simulink model "PSO_MPPT"  (R2018a)
settings: Solver=VariableStepAuto  StartTime=0.0  StopTime=10  FixedStep=1  RelTol=1e-3
libraries: powerlib x9, powerlib_meascontrol x2, re_lib x1
settings Model: Creator=Rodney Tan  LastModifiedBy=hp
settings SolverCC: ZeroCrossAlgorithm=Adaptive  AlgebraicLoopSolver=LineSearch
settings OptimizationCC: LifeSpan=inf
settings DebuggingCC: MaxConsecutiveZCsMsg=none  MaskedZcDiagnostic=none  IgnoredZcDiagnostic=none  SFUnexpectedBacktrackingDiag=warning  SFNoUnconditionalDefaultTransitionDiag=warning  SFExecutionAtInitializationDiag=none
settings CodeAppCC: StateflowObjectComments=on
settings GRTTargetCC: TargetLangStandard=C89/C90 (ANSI)  GeneratePreprocessorConditionals=Disable all
settings ConfigComp: CovMetricSettings=dw  CovHtmlReporting=on  CovSaveCumulativeToWorkspaceVar=on  CovSaveSingleToWorkspaceVar=on  CovExternalEMLEnable=off
settings SimscapeCC: SimscapeNormalizeSystem=off

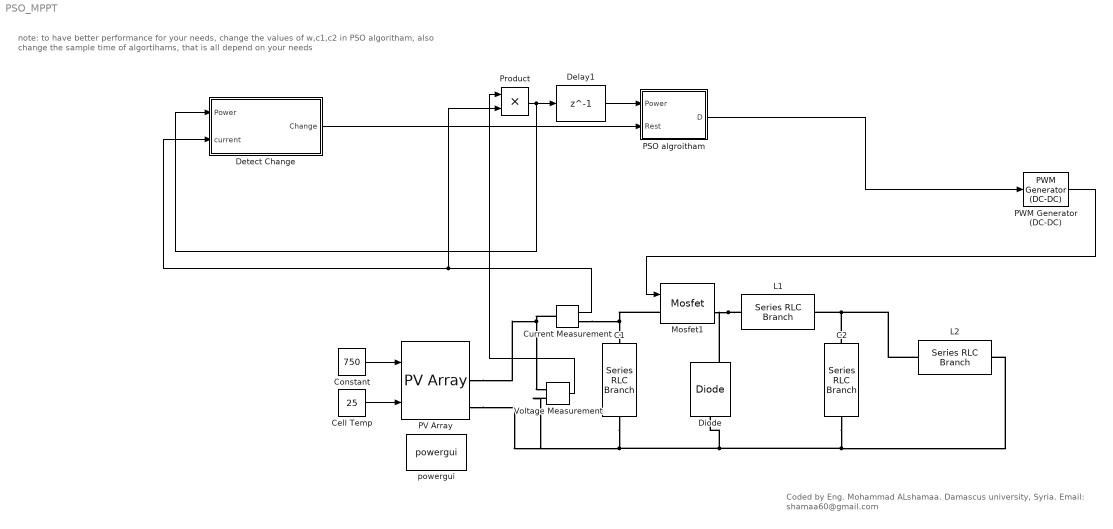
== system PSO_MPPT ==
  note: note: to have better performance for your needs,
      | change the values of w,c1,c2 in PSO algoritham, also change the sample time of algortihams, that is all depend on your needs
  note: Coded by Eng. Mohammad ALshamaa.
      | Damascus university, Syria.
      | Email: shamaa60@gmail.com
  " C2" : powerlib/Elements/Series RLC Branch  LConnTagsString=__new0  RConnTagsString=__new0  BranchType=C  Resistance=0.1  Inductance=1e-3  SetiL0=off  InitialCurrent=0  Capacitance=1000e-6  Setx0=off  InitialVoltage=0  Measurements=None
  C1 : powerlib/Elements/Series RLC Branch  LConnTagsString=__new0  RConnTagsString=__new0  BranchType=C  Resistance=0.1  Inductance=1e-3  SetiL0=off  InitialCurrent=0  Capacitance=1000e-6  Setx0=off  InitialVoltage=0  Measurements=None
  Cell Temp : Constant  Value=25
  Constant : Constant  Value=750
  Current Measurement : powerlib/Measurements/Current Measurement  PhasorSimulation=off  OutputType=Complex  PSBequivalent=0
  Delay1 : Delay  DelayLength=1  InputProcessing=Columns as channels (frame based)
  Detect Change : Subsystem
  Diode : powerlib/Power Electronics/Diode  Ron=0  Lon=0  Vf=0  IC=0  UseSnubber=0  Rs=500  Cs=250e-9  Measurements=on
  L1 : powerlib/Elements/Series RLC Branch  LConnTagsString=__new0  RConnTagsString=__new0  BranchType=L  Resistance=1  Inductance=20e-3  SetiL0=off  InitialCurrent=0  Capacitance=1e-6  Setx0=off  InitialVoltage=0  Measurements=None
  L2 : powerlib/Elements/Series RLC Branch  LConnTagsString=__new0  RConnTagsString=__new0  BranchType=R  Resistance=1  Inductance=10e-3  SetiL0=off  InitialCurrent=0  Capacitance=1e-6  Setx0=off  InitialVoltage=0  Measurements=None
  Mosfet1 : powerlib/Power Electronics/Mosfet  Ron=0  Lon=0  Rd=0  Vfd=0  IC=0  Rs=1e5  Cs=inf  Measurements=on
  PSO algroitham : MATLAB Function  TreatAsAtomicUnit=on  SystemSampleTime=0.05
  PV Array : re_lib/Solar/PV Array  Npar=1  Nser=1  PlotType=array @ 25 deg.C & specified irradiances  S_vec="[ 1000  750  100 ]"  Temp_C_vec="[ 45 25  ]"  ModuleName=1Soltech 1STH-215-P  PlotWhenSelected=off  Pm=213.15  Ncell=60  Voc=36.3  Isc=7.84  Vm=29  Im=7.35  beta_Voc_pc=-0.36099  alpha_Isc_pc=0.102  beta_Voc=-0.13104  alpha_Isc=0.007997  IL=7.8649  I0=2.9259e-10  nI=0.98117  Rsh=313.3991  Rs=0.39383  BAL=off  Tc=1e-6  Tfilter=5e-3
  PWM Generator (DC-DC) : powerlib_meascontrol/Pulse & Signal Generators/PWM Generator (DC-DC)  Fsw=10e3  Ts=0
  Product : Product
  Voltage Measurement : powerlib/Measurements/Voltage Measurement  PhasorSimulation=off  OutputType=Complex  PSBequivalent=0
  powergui : powerlib/powergui  Priority=1  SimulationMode=Continuous  SampleTime=1e-3  frequency=60  Iterations=50  frequencyindice=0  Pbase=100e6  ErrMax=1e-4  UnitsV=kV  UnitsW=MW  buscounter=0  FunctionMessages=off  echomessages=off  EnableUseOfTLC=off  CurrentSourceSwitches=off  DisableSnubberDevices=off  DisableRonSwitches=off  DisableVfSwitches=off  DisplayEquations=off  SolverType=Tustin/Backward Euler (TBE)  Interpol=off  ExternalGateDelay=off  methode=off  Ts=100  x0status=blocks  SPID=off  SwTol=0  HookPort=off  RestoreLinks=warning  ResistiveCurrentMeasurement=off  Frange=[0:2:500]  Ylog=off  Xlog=on  ShowGrid=off  save=off  variable=ZData  structure=0  ZoomFFT=off  StartTime=0.0  cycles=1  DisplayStyle=1  fundamental=60  FreqAxis=off  MaxFrequency=1000  frequencyindicesteady=1  RmsSteady=1  display=off
  wires:
  Cell Temp/1 -> PV Array/2
  Constant/1 -> PV Array/1
  PWM Generator (DC-DC)/1 -> Mosfet1/1
  Voltage Measurement/1 -> Product/1
  Delay1/1 -> PSO algroitham/1(Power)
  PSO algroitham/1(D) -> PWM Generator (DC-DC)/1
  Current Measurement/1 -> Detect Change/2(current), Product/2
  Product/1 -> Detect Change/1(Power), Delay1/1
  Detect Change/1(Change) -> PSO algroitham/2(Rest)
  connections:
  " C2"/LConn1 -- L2/LConn1 -- L1/RConn1
  " C2"/RConn1 -- L2/RConn1 -- Diode/LConn1 -- Voltage Measurement/LConn2 -- PV Array/RConn2 -- C1/RConn1
  L1/LConn1 -- Diode/RConn1 -- Mosfet1/RConn1
  Mosfet1/LConn1 -- Current Measurement/RConn1 -- C1/LConn1
  PV Array/RConn1 -- Current Measurement/LConn1 -- Voltage Measurement/LConn1

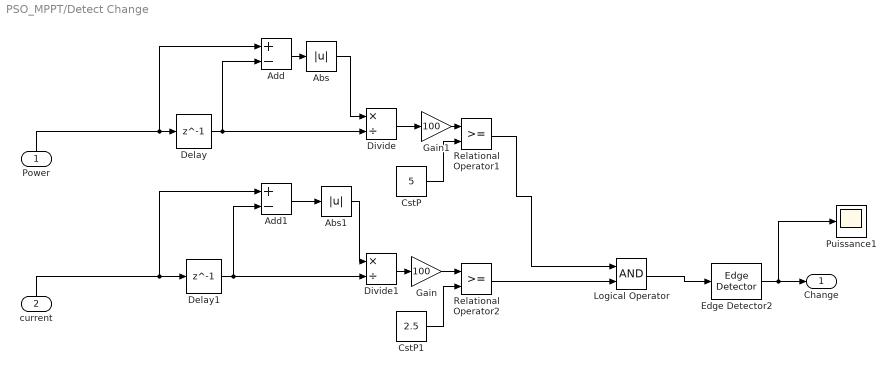
== system PSO_MPPT/Detect Change ==
  Power : Inport
  current : Inport  Port=2
  Abs : Abs
  Abs1 : Abs
  Add : Sum  Inputs=+-
  Add1 : Sum  Inputs=+-
  CstP : Constant  Value=5
  CstP1 : Constant  Value=2.5
  Delay : Delay  DelayLength=1
  Delay1 : Delay  DelayLength=1
  Divide : Product  Inputs=*/
  Divide1 : Product  Inputs=*/
  Edge Detector2 : powerlib_meascontrol/Logic/Edge Detector  model=Rising  ic=0  Ts=0
      settings: SourceProductName=Simscape Power Systems  SourceProductBaseCode=PS
  Gain : Gain  Gain=100
  Gain1 : Gain  Gain=100
  Logical Operator : Logic  AllPortsSameDT=off  OutDataTypeStr=boolean
  Puissance1 : Scope
  Relational Operator1 : RelationalOperator  OutDataTypeStr=boolean  RndMeth=Nearest
  Relational Operator2 : RelationalOperator  OutDataTypeStr=boolean  RndMeth=Nearest
  Change : Outport
  wires:
  Relational Operator1/1 -> Logical Operator/1
  Add/1 -> Abs/1
  Delay/1 -> Divide/2, Add/2
  Power/1 -> Add/1, Delay/1
  Abs/1 -> Divide/1
  CstP/1 -> Relational Operator1/2
  Logical Operator/1 -> Edge Detector2/1
  Delay1/1 -> Add1/2, Divide1/2
  CstP1/1 -> Relational Operator2/2
  current/1 -> Add1/1, Delay1/1
  Abs1/1 -> Divide1/1
  Add1/1 -> Abs1/1
  Relational Operator2/1 -> Logical Operator/2
  Divide1/1 -> Gain/1
  Gain/1 -> Relational Operator2/1
  Divide/1 -> Gain1/1
  Gain1/1 -> Relational Operator1/1
  Edge Detector2/1 -> Puissance1/1, Change/1

== matlab function PSO_MPPT/PSO algroitham ==
  settings: updateMethod=DISCRETE
  data: Power input; D output; Rest input
function D   = fcn(Power, Rest)
persistent particals
persistent pbest
persistent gbest
persistent velocity
persistent Dcurrent
persistent Powerbest
persistent u
persistent gpowerbest
persistent idx
persistent xx
if isempty(xx)
   xx=0; 
end
if isempty(particals) || (Rest==1 && xx==1)
particals=zeros(4,1); 
particals(1)=0.2;
particals(2)=0.3;
particals(3)=0.6;
particals(4)=0.9;
velocity=zeros(4,1)
pbest=zeros(4,1);
Powerbest=zeros(4,1);
gbest=0.5;
Dcurrent=0;
gpowerbest=0;
u=0;
idx=0;
end
if sum(abs(velocity))>0.017 || sum(abs(velocity))==0
u=u+1;
if(u==6)
    u=1;
end
if u>1 && u<=5
    if Power>Powerbest(u-1)
    Powerbest(u-1)=Power;
       pbest(u-1)=Dcurrent;
    end
end
if (u>=1 && u<=4)
   D=particals(u);
   Dcurrent=particals(u);
elseif (u==5)
    [gpowerbest,idx] = max(Powerbest);
    gbest=pbest(idx);
    D=gbest;
    velocity(1)=updatevelocity(velocity(1),pbest(1),particals(1),gbest)
    velocity(2)=updatevelocity(velocity(2),pbest(2),particals(2),gbest)
    velocity(3)=updatevelocity(velocity(3),pbest(3),particals(3),gbest)
    velocity(4)=updatevelocity(velocity(4),pbest(4),particals(4),gbest)
    particals(1)=updateduty(particals(1),velocity(1))
    particals(2)=updateduty(particals(2),velocity(2))
    particals(3)=updateduty(particals(3),velocity(3))
    particals(4)=updateduty(particals(4),velocity(4))
else
   D=0;
end
else
    D=gbest;
    xx=1;
end
end


function vfinal=updatevelocity(velocity,pobest,d,gwbest)
w=0.4;
c1=1.025;   
c2=1.025;         
vfinal = (w*velocity)+(c1*rand(1)*(pobest-d))+(c2*rand(1)*(gwbest-d));
end
function dfinal=updateduty(d,velocity)
dup=d+velocity;
if(dup>1)
    dfinal=1;
elseif(dup<0)
    dfinal=0;
else
    dfinal=dup;
end
end
